simulink model "Dynamic_model"  (R2021b)
settings: Solver=VariableStepAuto  StartTime=0.0  StopTime=5  RelTol=1e-3
StopFcn:
  | clc
  | 
  | pos_n=pos.signals.values;
  | Joint_pxn=join_px.signals.values;
  | Joint_pyn=join_py.signals.values;
  | Joint_pzn=join_pz.signals.values;
  | 
  | xe=pos_n(:,1);
  | ye=pos_n(:,2);
  | ze=pos_n(:,3);
  | for i=1:size(pos_n,1)
  | figure(1)
  | clf
  | plot3(xe(1:i),ye(1:i),ze(1:i),'b--','LineWidth',2)
  | hold on
  | plot3(Joint_pxn(i,:),Joint_pyn(i,:),Joint_pzn(i,:),'r-o','LineWidth',2,'MarkerFaceColor','g','MarkerSize',7)
  | view(56,48)
  | 
  | grid on
  | pause(0.1)
  | end
  | 
  | xlabel('x(m)')
  | ylabel('y(m)')
  | zlabel('z(m)')
settings Model: Creator=HJokar  LastModifiedBy=pc
settings SolverCC: AlgebraicLoopSolver=TrustRegion
settings DataIOCC: ReturnWorkspaceOutputs=off
settings DebuggingCC: SFMachineParentedDataDiag=warning  ArithmeticOperatorsInVariantConditions=warning
settings SFSimCC: CustomCodeUndefinedFunction=UseInterfaceOnly

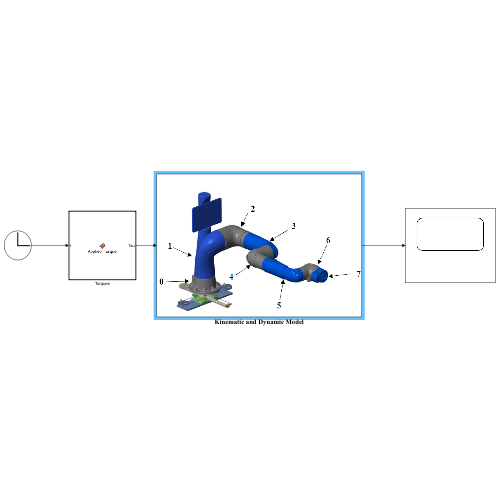
[thumbnail: Simulink's stored preview of the top-level diagram]
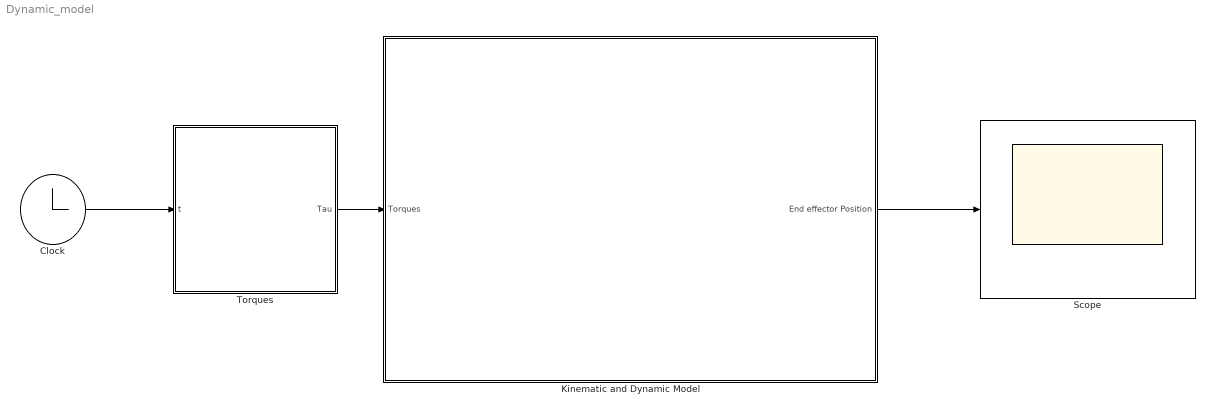
== system Dynamic_model ==
  Clock : Clock
  Kinematic and Dynamic Model : Subsystem
      mask Display: image('robotfig.png');
  Scope : Scope
  Torques : MATLAB Function  TreatAsAtomicUnit=on
  wires:
  Clock/1 -> Torques/1(t)
  Torques/1(Tau) -> Kinematic and Dynamic Model/1(Torques)
  Kinematic and Dynamic Model/1(End effector Position) -> Scope/1

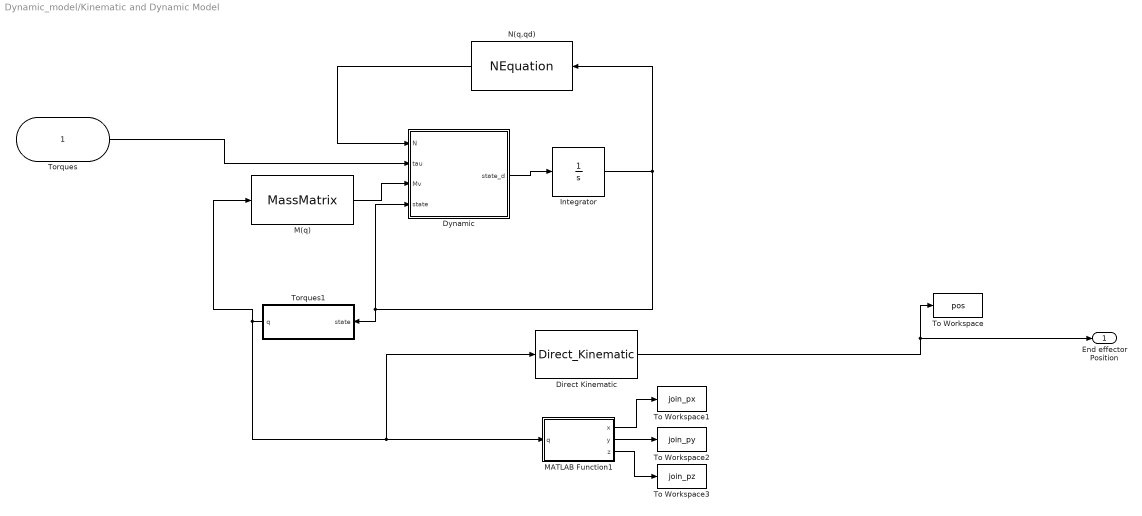
== system Dynamic_model/Kinematic and Dynamic Model ==
  Torques : Inport
  Direct Kinematic : MATLABFcn  MATLABFcn=Direct_Kinematic  OutputSignalType=real
  Dynamic : MATLAB Function  TreatAsAtomicUnit=on
  Integrator : Integrator  InitialCondition=zeros(14,1)
  M(q) : MATLABFcn  MATLABFcn=MassMatrix  OutputSignalType=real
  MATLAB Function1 : MATLAB Function  TreatAsAtomicUnit=on
  N(q,qd) : MATLABFcn  MATLABFcn=NEquation  OutputSignalType=real
  To Workspace : ToWorkspace  VariableName=pos  SaveFormat=Structure With Time  SampleTime=-1
  To Workspace1 : ToWorkspace  VariableName=join_px  SaveFormat=Structure With Time  SampleTime=-1
  To Workspace2 : ToWorkspace  VariableName=join_py  SaveFormat=Structure With Time  SampleTime=-1
  To Workspace3 : ToWorkspace  VariableName=join_pz  SaveFormat=Structure With Time  SampleTime=-1
  Torques1 : MATLAB Function  TreatAsAtomicUnit=on
  End effector Position : Outport  VectorParamsAs1DForOutWhenUnconnected=off
  wires:
  MATLAB Function1/3(z) -> To Workspace3/1
  M(q)/1 -> Dynamic/3(Mv)
  Torques/1 -> Dynamic/2(tau)
  Torques1/1(q) -> M(q)/1, Direct Kinematic/1, MATLAB Function1/1(q)
  Direct Kinematic/1 -> End effector Position/1, To Workspace/1
  N(q,qd)/1 -> Dynamic/1(N)
  Dynamic/1(state_d) -> Integrator/1
  MATLAB Function1/1(x) -> To Workspace1/1
  Integrator/1 -> N(q,qd)/1, Dynamic/4(state), Torques1/1(state)
  MATLAB Function1/2(y) -> To Workspace2/1

== matlab function Dynamic_model/Kinematic and Dynamic Model/Dynamic ==
  data: N input; state_d output; tau input; Mv input; state input
function  state_d= Dynamic_model(N,tau,Mv,state)
nL=7;
state_d=zeros(2*nL,1);
q=state(1:nL);
qd=state(nL+1:2*nL);
M=reshape(Mv,[nL,nL]);
%=============== Dynamic ====================
qdd=M^(-1)*(tau-N);
state_d(1:nL)=qd;
state_d(nL+1:2*nL)=qdd;
end

== matlab function Dynamic_model/Torques ==
  data: Tau output; t input
function Tau  = Applied_Torque(t)
Tau=zeros(7,1);
Tau(1)=0;
Tau(2)=0;
Tau(3)=0;
Tau(4)=0;
Tau(5)=0;
Tau(6)=0;
Tau(7)=0;

== matlab function Dynamic_model/Kinematic and Dynamic Model/Torques1 ==
  data: q output; state input
function q  = fcn(state)
nL=7;
q=state(1:nL);

== matlab function Dynamic_model/Kinematic and Dynamic Model/MATLAB Function1 ==
  data: q input; x output; y output; z output
function [x,y,z]=Frame_origin(q)

nL=7;
d=[317*cos(asin(81/317)) 194.5 400 168.5 400 136.3 134.75]'*1e-3;
a=[0 81 0 0 0 0 0]'*1e-3; 
alpha=[0 -pi/2 -pi/2 -pi/2 pi/2 pi/2 -pi/2]';
teta=q;
teta(2)=teta(2)-pi/2;
Ti_im={zeros(4,4),zeros(4,4),zeros(4,4),zeros(4,4),zeros(4,4),zeros(4,4),zeros(4,4)};
Ti=Ti_im;
for i = 1:nL
    Ti_im{i} =[ cos(teta(i)) -sin(teta(i)) 0 a(i);
        sin(teta(i))*cos(alpha(i)) cos(teta(i))*cos(alpha(i)) -sin(alpha(i)) -sin(alpha(i))*d(i);
        sin(teta(i))*sin(alpha(i)) cos(teta(i))*sin(alpha(i)) cos(alpha(i)) cos(alpha(i))*d(i);
        0 0 0 1];
end
% 0_T_i
for i = 1:nL
    if i==1
        Ti{i}=Ti_im{i};
        
    else
        Ti{i}=Ti{i-1}*Ti_im{i};
    end
end
% Robot Configuration:

x=[0,Ti{1}(1,4) Ti{2}(1,4) Ti{3}(1,4) Ti{4}(1,4) Ti{5}(1,4) Ti{6}(1,4) Ti{7}(1,4)]';
y=[0,Ti{1}(2,4) Ti{2}(2,4) Ti{3}(2,4) Ti{4}(2,4) Ti{5}(2,4) Ti{6}(2,4) Ti{7}(2,4)]';
z=[0,Ti{1}(3,4) Ti{2}(3,4) Ti{3}(3,4) Ti{4}(3,4) Ti{5}(3,4) Ti{6}(3,4) Ti{7}(3,4)]';
end
